simulink model "chuanji"  (Simulink 7.3)
settings: Solver=ode45  StartTime=0.0  StopTime=150.0  RelTol=1e-3
libraries: simulink_extras x2
settings Model: Creator=CETC  LastModifiedBy=Administrator
settings DebuggingCC: SolverPrmCheckMsg=none  StrictBusMsg=ErrorLevel1

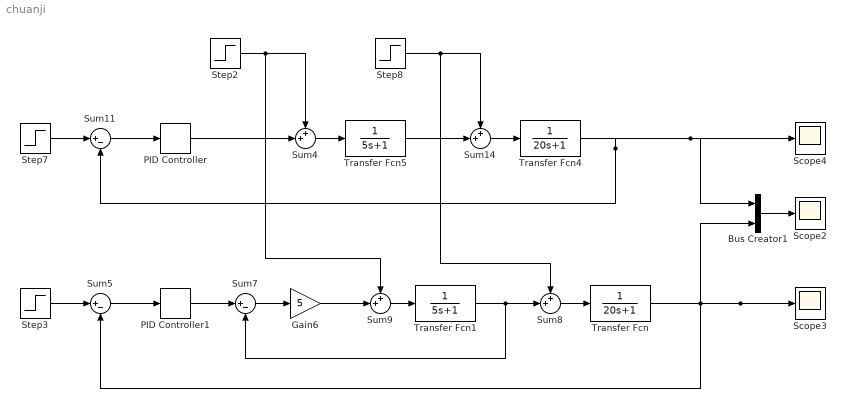
== system chuanji ==
  Bus Creator1 : BusCreator  Inputs=2
  Gain6 : Gain  Gain=5  ParameterDataType=fixdt(1, 16)  ParameterScaling=2^0  OutDataType=fixdt(1, 16)  OutScaling=2^0
  PID Controller : simulink_extras/Additional Linear/PID Controller  SystemSampleTime=-1  P=9  I=1  D=2
  PID Controller1 : simulink_extras/Additional Linear/PID Controller  SystemSampleTime=-1  P=9  I=1  D=2
  Scope2 : Scope
  Scope3 : Scope
      settings: SaveName=ScopeData2
  Scope4 : Scope
      settings: SaveName=ScopeData3
  Step2 : Step  Time=60  SampleTime=0
  Step3 : Step  Time=0  SampleTime=0
  Step7 : Step  Time=0  SampleTime=0
  Step8 : Step  Time=60  After=0  SampleTime=0
  Sum11 : Sum  Inputs=|+-  OutDataType=fixdt(1, 16)  OutScaling=2^0
  Sum{4,8..9,14} (4 alike) : Sum  Inputs=++|  OutDataType=fixdt(1, 16)  OutScaling=2^0
  Sum5 : Sum  Inputs=|+-  OutDataType=fixdt(1, 16)  OutScaling=2^0
  Sum7 : Sum  Inputs=|+-  OutDataType=fixdt(1, 16)  OutScaling=2^0
  Transfer Fcn : TransferFcn  Denominator=[20 1]
  Transfer Fcn1 : TransferFcn  Denominator=[5 1]
  Transfer Fcn4 : TransferFcn  Denominator=[20 1]
  Transfer Fcn5 : TransferFcn  Denominator=[5 1]
  wires:
  Step3/1 -> Sum5/1
  Sum5/1 -> PID Controller1/1
  PID Controller1/1 -> Sum7/1
  Sum7/1 -> Gain6/1
  Transfer Fcn1/1 -> Sum8/2, Sum7/2
  Sum8/1 -> Transfer Fcn/1
  Sum9/1 -> Transfer Fcn1/1
  Gain6/1 -> Sum9/2
  Step7/1 -> Sum11/1
  Sum11/1 -> PID Controller/1
  PID Controller/1 -> Sum4/2
  Transfer Fcn5/1 -> Sum14/2
  Sum14/1 -> Transfer Fcn4/1
  Step8/1 -> Sum14/1, Sum8/1
  Transfer Fcn4/1 -> Sum11/2, Scope4/1, Bus Creator1/1
  Transfer Fcn/1 -> Sum5/2, Scope3/1, Bus Creator1/2
  Bus Creator1/1 -> Scope2/1
  Step2/1 -> Sum4/1, Sum9/1
  Sum4/1 -> Transfer Fcn5/1
